simulink model "tclab_temp_control"  (R2021a)
settings: Solver=VariableStepAuto  StartTime=0.0  StopTime=500  RelTol=1e-3  EnableMultiTasking=on
StartFcn:
  | clear all
libraries: adrc_toolbox_library x2, realtime_pacer_lib x1
settings Model: Creator=johnh  LastModifiedBy=PC
settings SolverCC: AlgebraicLoopSolver=TrustRegion
settings DataIOCC: ReturnWorkspaceOutputs=off
settings OptimizationCC: LifeSpan=inf
settings DebuggingCC: SFUnexpectedBacktrackingDiag=warning  SFNoUnconditionalDefaultTransitionDiag=warning  SFExecutionAtInitializationDiag=none  SFMachineParentedDataDiag=warning  ArithmeticOperatorsInVariantConditions=warning
settings SFSimCC: SimUseLocalCustomCode=off  CustomCodeUndefinedFunction=UseInterfaceOnly
settings RTWCC: RTWUseLocalCustomCode=off
settings CodeAppCC: StateflowObjectComments=on
settings GRTTargetCC: TargetLangStandard=C89/C90 (ANSI)
settings ConfigComp: CovMetricSettings=dw  CovSaveCumulativeToWorkspaceVar=on  CovSaveSingleToWorkspaceVar=on  CovExternalEMLEnable=off

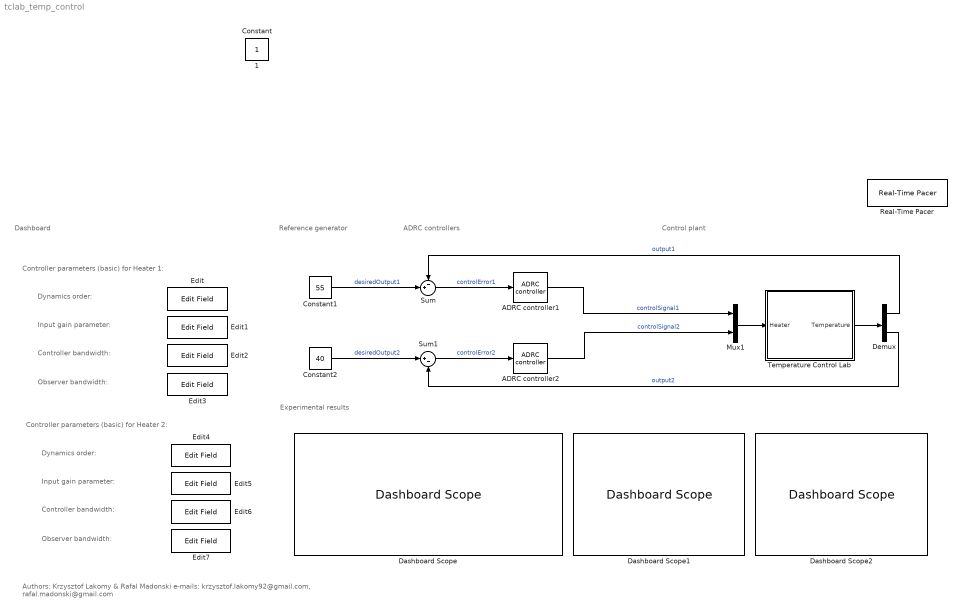
== system tclab_temp_control ==
  note: Observer bandwidth:
  note: Controller bandwidth:
  note: Authors: Krzysztof Lakomy & Rafal Madonski
      | e-mails: krzysztof.lakomy92@gmail.com, rafal.madonski@gmail.com
  note: Experimental results
  note: Dashboard
  note: ADRC controllers
  note: Dynamics order:
  note: Control plant
  note: Input gain parameter:
  note: Controller parameters (basic) for Heater 1:
  note: Reference
      | generator
  note: Controller parameters (basic) for Heater 2:
  note: Input gain parameter:
  note: Dynamics order:
  note: Controller bandwidth:
  note: Observer bandwidth:
  ADRC controller1 : adrc_toolbox_library/ADRC controller  dynamicsOrder=1  controllerBandwidth=3  controllerBandwidthSource=Internal  observerBandwidth=10  observerBandwidthSource=Internal  inputGainParameter=5  inputGainSource=Internal  saturationEnabled=on  UpperLimit=100  LowerLimit=0  antiPeakingEnabled=off  antiPeakingTime=0.2
      link override State feedback robust controller/Saturation: VariantControlMode=label  LabelModeActiveChoice=saturation_off
      settings: SourceProductName=ADRC toolbox
  ADRC controller2 : adrc_toolbox_library/ADRC controller  dynamicsOrder=1  controllerBandwidth=3  controllerBandwidthSource=Internal  observerBandwidth=10  observerBandwidthSource=Internal  inputGainParameter=5  inputGainSource=Internal  saturationEnabled=on  UpperLimit=100  LowerLimit=0  antiPeakingEnabled=off  antiPeakingTime=0.2
      link override State feedback robust controller/Saturation: VariantControlMode=label  LabelModeActiveChoice=saturation_off
      settings: SourceProductName=ADRC toolbox
  Constant1 : Constant  Value=55
  Constant2 : Constant  Value=40
  Dashboard Scope : DashboardScope  Ymin=0  Ymax=100
  Dashboard Scope1 : DashboardScope  Ymin=0  Ymax=100
  Dashboard Scope2 : DashboardScope  Ymin=-50  Ymax=50
  Demux : Demux  Outputs=2
  Edit{,1..7} (8 alike) : EditField  LabelPosition=Hide  ShowInitialText=on  Alignment=Center
  Mux1 : Mux  Inputs=2
  Real-Time Pacer : realtime_pacer_lib/Real-Time Pacer  simTimePerRealTime=1
  Sum : Sum  Inputs=-+|
  Sum1 : Sum  Inputs=|+-
  Temperature Control Lab : Subsystem
      mask Display: image('tclab.png');
  1 : Constant  IOType=siggen
  Constant : Constant  IOType=siggen
  wires:
  Demux/1 -> Sum/1  "output1"
  Constant1/1 -> Sum/2  "desiredOutput1"
  ADRC controller1/1 -> Mux1/1  "controlSignal1"
  Sum/1 -> ADRC controller1/1  "controlError1"
  Temperature Control Lab/1(Temperature) -> Demux/1
  Mux1/1 -> Temperature Control Lab/1(Heater)
  ADRC controller2/1 -> Mux1/2  "controlSignal2"
  Sum1/1 -> ADRC controller2/1  "controlError2"
  Constant2/1 -> Sum1/1  "desiredOutput2"
  Demux/2 -> Sum1/2  "output2"

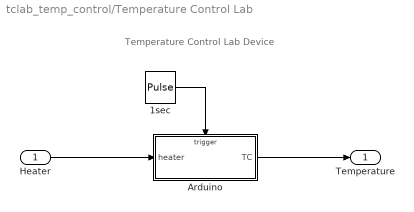
== system tclab_temp_control/Temperature Control Lab ==
  note: Temperature Control Lab Device
  Heater : Inport
  1sec : DiscretePulseGenerator  PulseType=Time based  Period=1  PulseWidth=50
  Arduino : Subsystem  TreatAsAtomicUnit=on
  Temperature : Outport  VectorParamsAs1DForOutWhenUnconnected=off
  wires:
  1sec/1 -> Arduino/Trigger
  Arduino/1(TC) -> Temperature/1
  Heater/1 -> Arduino/1(heater)

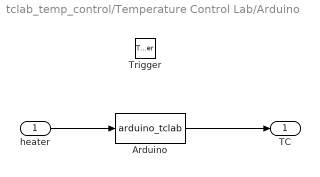
== system tclab_temp_control/Temperature Control Lab/Arduino ==
  heater : Inport  LatchByDelayingOutsideSignal=on
  Trigger : TriggerPort  VariantControl=Variant
  Arduino : MATLABFcn  MATLABFcn=arduino_tclab
  TC : Outport  InitialOutput=[23 23]  VectorParamsAs1DForOutWhenUnconnected=off
  wires:
  heater/1 -> Arduino/1
  Arduino/1 -> TC/1
